simulink model "LAB1_1_real"  (R2025b)
settings: Solver=ode3  StartTime=0.0  StopTime=10  FixedStep=0.001  RelTol=1e-3
undefined symbols (not defined in the file or in its folder): BEMF_comp, daq, den_Hi, Fri_comp, In_comp, Kd, Ki, Kp, Kw, mot, National_Instruments, num_Hi, om_comp, PCI, sens, Tausf, Tl
libraries: sldrtlib x3, simulink x1
settings Model: SimulationMode=external  ExtModeTrigDuration=100001  Creator=delpratogi  LastModifiedBy=Simone
settings DataIOCC: ReturnWorkspaceOutputs=off
settings HardwareCC: ProdBitPerLong=64.0  ProdHWDeviceType=Intel->x86-64 (Linux 64)
settings RTWCC: SystemTargetFile=sldrt.tlc  TemplateMakefile=sldrt.tmf  RTWCompilerOptimization=on  Description=Simulink Desktop Real-Time
settings CodeAppCC: MaxIdLength=95.0
settings STFCustomTargetCC: SystemTargetFile=sldrt.tlc  TargetLangStandard=C99 (ISO)  ModelReferenceCompliant=off  ConcurrentExecutionCompliant=off  MATLABClassNameForMDSCustomization=Simulink.SoftwareTarget.TargetSpecificTriggerConfigurationBase

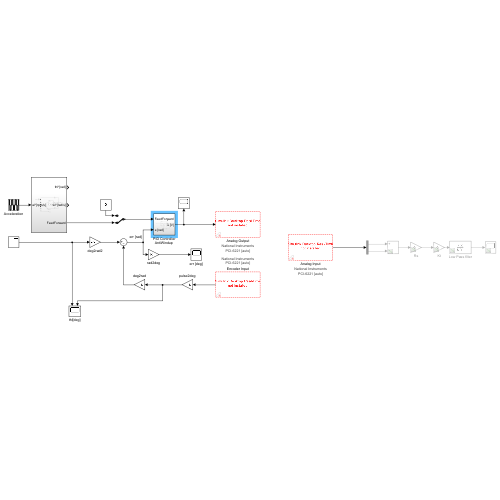
[thumbnail: Simulink's stored preview of the top-level diagram]
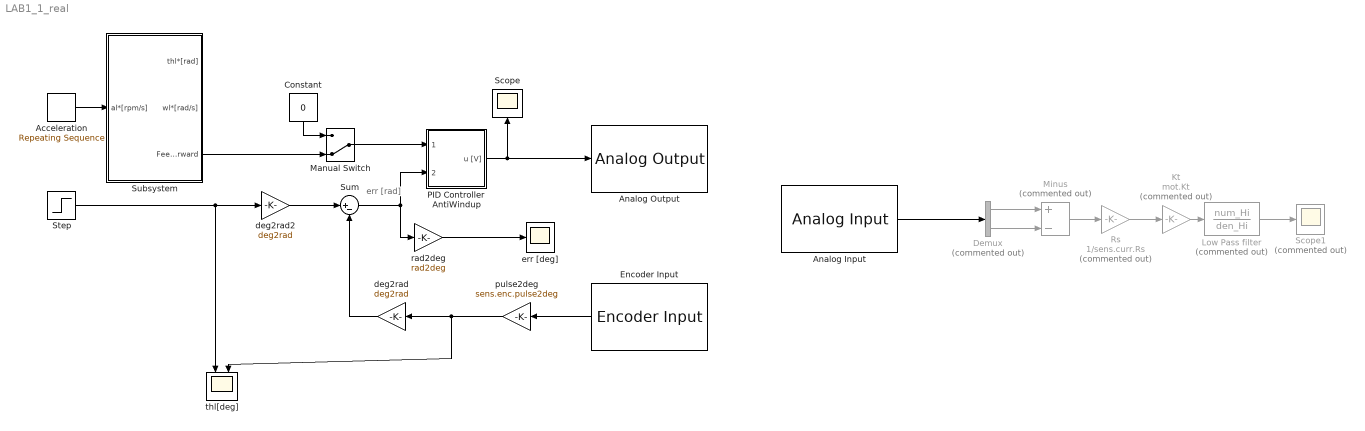
== system LAB1_1_real ==
  note: err [rad]
  Acceleration : simulink/Sources/Repeating Sequence  rep_seq_t=[0, 0.5, 0.50001, 1, 1.0001, 2, 2.0001, 2.5, 2.50001, 3]  rep_seq_y=[900, 900, 0, 0, -900, -900, 0, 0, 900, 900]
  Analog Input : sldrtlib/Analog Input  SampleTime=0.001  MaxMissedTicks=10  ShowMissedTicks=off  YieldWhenWaiting=off  DrvName=National_Instruments/PCI-6221  DrvAddress=4294967295  DrvOptions=[0 0 0 2 0]  Channels=[1,2]  RangeMode=1  VoltRange=1  DataType=1
      settings: AttributesFormatString=National Instruments\nPCI-6221 [auto]
  Analog Output : sldrtlib/Analog Output  SampleTime=0.001  MaxMissedTicks=10  ShowMissedTicks=off  YieldWhenWaiting=off  DrvName=National_Instruments/PCI-6221  DrvAddress=4294967295  DrvOptions=[0 0 0 2 0]  Channels=1  RangeMode=1  VoltRange=1  InitialValue=0  FinalValue=0
      settings: AttributesFormatString=National Instruments\nPCI-6221 [auto]
  Constant : Constant  Value=0
  Demux : Demux  Commented=on  Outputs=2
  Encoder Input : sldrtlib/Encoder Input  SampleTime=0.001  MaxMissedTicks=10  ShowMissedTicks=off  YieldWhenWaiting=off  DrvName=National_Instruments/PCI-6221  DrvAddress=4294967295  DrvOptions=[0 0 0 2 0]  Channels=1  QuadMode=3  IndexPulse=1  InputFilter=Inf  DataType=1
      settings: AttributesFormatString=National Instruments\nPCI-6221 [auto]
  Kt : Gain  Commented=on  Gain=mot.Kt
  Low Pass filter : TransferFcn  Commented=on  Numerator=num_Hi  Denominator=den_Hi
  Manual Switch : ManualSwitch  CurrentSetting=0
  Minus : Sum  Commented=on  Inputs=+-
  "PID Controller AntiWindup " : Subsystem
  Rs : Gain  Commented=on  Gain=1/sens.curr.Rs
  Scope : Scope
      settings: ActiveDisplayYMinimum=-2.61034  ActiveDisplayYMaximum=11.40115
  Scope1 : Scope  Commented=on
  Step : Step  Time=0  After=360  SampleTime=0
  Subsystem : Subsystem
  Sum : Sum  Inputs=|+-
  deg2rad : Gain  Gain=deg2rad
  deg2rad2 : Gain  Gain=deg2rad
  err [deg] : Scope
      settings: ActiveDisplayYMinimum=-346.32  ActiveDisplayYMaximum=438.48  DataLoggingVariableName=ScopeData2
  pulse2deg : Gain  Gain=sens.enc.pulse2deg
  rad2deg : Gain  Gain=rad2deg
  thl[deg] : Scope  NumInputPorts=2
      settings: ActiveDisplayYMinimum=-78.48  ActiveDisplayYMaximum=706.32
  wires:
  Analog Input/1 -> Demux/1
  Demux/1 -> Minus/1
  Encoder Input/1 -> pulse2deg/1
  Minus/1 -> Rs/1
  Demux/2 -> Minus/2
  Rs/1 -> Kt/1
  Low Pass filter/1 -> Scope1/1
  Kt/1 -> Low Pass filter/1
  pulse2deg/1 -> thl[deg]/2, deg2rad/1
  "PID Controller AntiWindup "/1(u [V]) -> Analog Output/1, Scope/1
  Sum/1 -> rad2deg/1, "PID Controller AntiWindup "/2(e [rad])
  deg2rad/1 -> Sum/2
  Step/1 -> thl[deg]/1, deg2rad2/1
  rad2deg/1 -> err [deg]/1
  deg2rad2/1 -> Sum/1
  Acceleration/1 -> Subsystem/1(al*[rpm/s])
  Subsystem/3(FeedForward) -> Manual Switch/2
  Manual Switch/1 -> "PID Controller AntiWindup "/1(FeedForward)
  Constant/1 -> Manual Switch/1

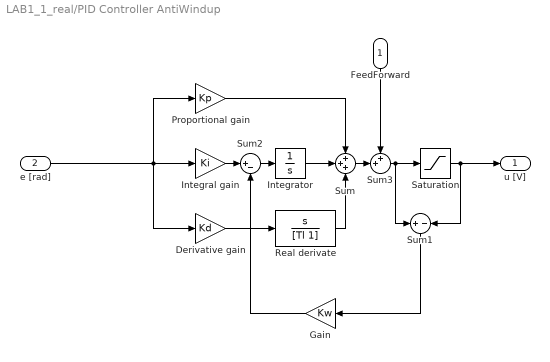
== system LAB1_1_real/PID Controller AntiWindup  ==
  FeedForward : Inport
  e [rad] : Inport  Port=2
  Derivative gain : Gain  Gain=Kd
  Gain : Gain  Gain=Kw
  "Integral gain " : Gain  Gain=Ki
  Integrator : Integrator
  Proportional gain : Gain  Gain=Kp
  Real derivate : TransferFcn  Numerator=[1 0]  Denominator=[Tl 1]
  Saturation : Saturate  UpperLimit=daq.dac.fs  LowerLimit=-daq.dac.fs
  Sum : Sum  Inputs=+++
  Sum1 : Sum  Inputs=+|-
  Sum2 : Sum  Inputs=|+-
  Sum3 : Sum  Inputs=++|
  u [V] : Outport
  wires:
  Real derivate/1 -> Sum/3
  Integrator/1 -> Sum/2
  e [rad]/1 -> Proportional gain/1, Derivative gain/1, "Integral gain "/1
  Proportional gain/1 -> Sum/1
  Derivative gain/1 -> Real derivate/1
  Saturation/1 -> Sum1/2, u [V]/1
  Sum1/1 -> Gain/1
  "Integral gain "/1 -> Sum2/1
  Sum2/1 -> Integrator/1
  Gain/1 -> Sum2/2
  Sum3/1 -> Sum1/1, Saturation/1
  Sum/1 -> Sum3/2
  FeedForward/1 -> Sum3/1

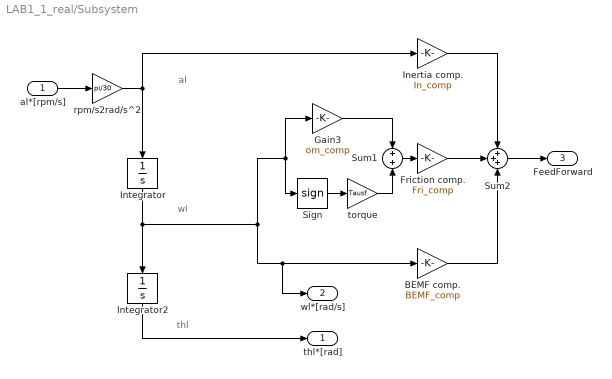
== system LAB1_1_real/Subsystem ==
  note: al
  note: wl
  note: thl
  al*[rpm/s] : Inport
  BEMF comp. : Gain  Gain=BEMF_comp
  Friction comp. : Gain  Gain=Fri_comp
  Gain3 : Gain  Gain=om_comp
  Inertia comp. : Gain  Gain=In_comp
  Integrator : Integrator
  Integrator2 : Integrator
  Sign : Signum  ZeroCross=off
  Sum1 : Sum
  Sum2 : Sum  Inputs=+++
  rpm/s2rad/s^2 : Gain  Gain=pi/30
  torque : Gain  Gain=Tausf
  thl*[rad] : Outport
  wl*[rad/s] : Outport  Port=2
  FeedForward : Outport  Port=3
  wires:
  Sign/1 -> torque/1
  torque/1 -> Sum1/2
  rpm/s2rad/s^2/1 -> Inertia comp./1, Integrator/1
  Gain3/1 -> Sum1/1
  Integrator2/1 -> thl*[rad]/1
  BEMF comp./1 -> Sum2/3
  al*[rpm/s]/1 -> rpm/s2rad/s^2/1
  Sum2/1 -> FeedForward/1
  Integrator/1 -> wl*[rad/s]/1, BEMF comp./1, Sign/1, Gain3/1, Integrator2/1
  Inertia comp./1 -> Sum2/1
  Friction comp./1 -> Sum2/2
  Sum1/1 -> Friction comp./1
